simulink library "aerolibgravity2"  (Simulink 6.0)
settings: Solver=ode45  SolverMode=SingleTasking  StartTime=0.0  StopTime=10.0  RelTol=1e-3
values from neighbouring files (symbols this model uses):
  s = aeroliblist    [asbhelp.m]
undefined symbols (not defined in the file or in its folder): aeroassertmsg, c, cd, epoch, fm, fn, k, m, maxdef, snorm
libraries: simulink x9, aerolibconvert x8, aerolibutil x2
(part 2 of 2)

== system aerolibgravity2/World Magnetic Model 2000/geomg1/Compute magnetic vector in spherical coordinates/For Iterator Subsystem/Time adjust the gauss coefficients ==
  n : Inport  LatchInput=off
  m : Inport  Port=2  LatchInput=off
  dt : Inport  Port=3  LatchInput=off
  Enable : EnablePort
  Assignment : Assignment  InputType=Matrix  RowSrc=External  ColumnSrc=External  DiagnosticForDimensions=Error
  Bus Creator : BusCreator  DialogController=Simulink.DDGSource_Bus  Inputs=5
  Bus Selector1 : BusSelector  DialogController=Simulink.DDGSource_Bus  OutputSignals=signal1,signal2,signal3,signal4,signal5
  Demux2 : Demux  Outputs=3
  If Action Subsystem : Subsystem  TreatAsAtomicUnit=on  PropExecContextAcrossSSBoundary=on
  Mux1 : Mux  Inputs=3
  Sum2 : Sum  Inputs=|++  SaturateOnIntegerOverflow=on
  Unit Delay : UnitDelay  Orientation=left  X0=zeros(maxdef+1,maxdef+1)  SampleTime=-1
  c[maxdef][maxdef] : Constant  Value=c
  cd[maxdef][maxdef] : Constant  Value=cd
  if (m~=0) : Subsystem  PropExecContextAcrossSSBoundary=on
  tc[13][13] : Outport
  wires:
  Sum2/1 -> tc[13][13]/1
  Unit Delay/1 -> Assignment/1
  if (m~=0)/1(tc[13][13]) -> Sum2/2
  Bus Selector1/4 -> If Action Subsystem/4(c)  "<signal4>"
  Bus Creator/1 -> Bus Selector1/1, if (m~=0)/1(bus)
  Demux2/3 -> Assignment/4
  Demux2/2 -> Assignment/3
  Demux2/1 -> Assignment/2
  Mux1/1 -> Demux2/1
  If Action Subsystem/3(col) -> Mux1/3
  If Action Subsystem/2(row) -> Mux1/2
  If Action Subsystem/1(tc) -> Mux1/1
  Assignment/1 -> Sum2/1, Unit Delay/1
  cd[maxdef][maxdef]/1 -> Bus Creator/5
  c[maxdef][maxdef]/1 -> Bus Creator/4
  dt/1 -> Bus Creator/3
  n/1 -> Bus Creator/2
  Bus Selector1/5 -> If Action Subsystem/5(cd)  "<signal5>"
  Bus Selector1/3 -> If Action Subsystem/3(dt)  "<signal3>"
  Bus Selector1/2 -> If Action Subsystem/2(n)  "<signal2>"
  Bus Selector1/1 -> If Action Subsystem/1(m)  "<signal1>"
  m/1 -> Bus Creator/1

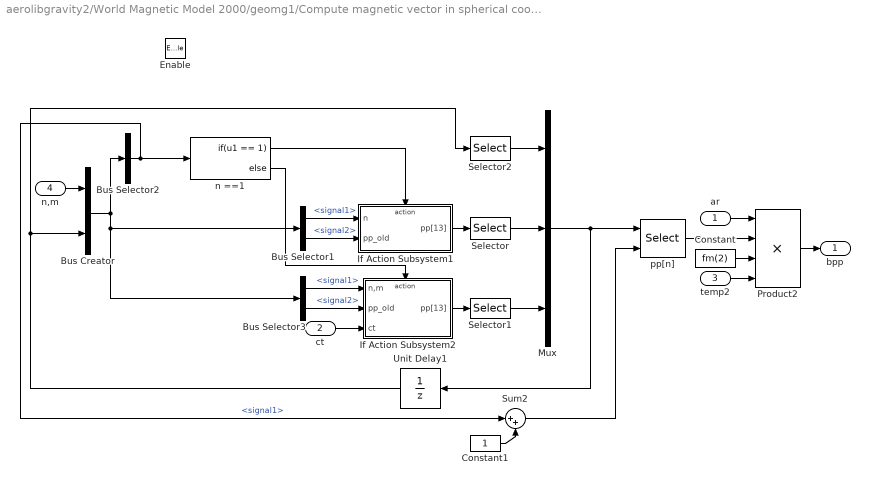
== system aerolibgravity2/World Magnetic Model 2000/geomg1/Compute magnetic vector in spherical coordinates/For Iterator Subsystem/Accumulate terms of the  spherical harmonic expansion/Special case - North/South Geographic Pole ==
  ar : Inport  LatchInput=off
  ct : Inport  Port=2  LatchInput=off
  temp2 : Inport  Port=3  LatchInput=off
  n,m : Inport  Port=4  LatchInput=off
  Enable : EnablePort
  Bus Creator : BusCreator  DialogController=Simulink.DDGSource_Bus  Inputs=2
  Bus Selector1 : BusSelector  DialogController=Simulink.DDGSource_Bus  OutputSignals=signal1.signal1,signal2
  Bus Selector2 : BusSelector  DialogController=Simulink.DDGSource_Bus  OutputSignals=signal1.signal1
  Bus Selector3 : BusSelector  DialogController=Simulink.DDGSource_Bus  OutputSignals=signal1,signal2
  Constant : Constant  Value=fm(2)
  Constant1 : Constant
  If Action Subsystem1 : Subsystem  AncestorBlock=|  PropExecContextAcrossSSBoundary=on
      | aerolibatmosratios/WMM 2000/geomg1/Compute magnetic vector in
      | spherical coordinates/For Iterator
      | Subsystem/Accumulate terms of the 
      | spherical harmonic expansion/Special case - North//South Geographic Pole/if (m~=0)/If Action
      | Subsystem1
  If Action Subsystem2 : Subsystem  AncestorBlock=|  PropExecContextAcrossSSBoundary=on
      | aerolibatmosratios/WMM 2000/geomg1/Compute magnetic vector in
      | spherical coordinates/For Iterator
      | Subsystem/Accumulate terms of the 
      | spherical harmonic expansion/Special case - North//South Geographic Pole/if (m~=0)/If Action
      | Subsystem2
  Mux : Mux  Inputs=3
  Product2 : Product  Inputs=4  SaturateOnIntegerOverflow=on
  Selector : Selector  Elements=[2]  Rows=[1 2]  Columns=-1  InputPortWidth=maxdef+1
  Selector1 : Selector  Elements=3:maxdef+1  InputPortWidth=maxdef+1
  Selector2 : Selector  Elements=[1]  Rows=[1 2]  Columns=-1  InputPortWidth=maxdef+1
  Sum2 : Sum  Inputs=|++  SaturateOnIntegerOverflow=on
  Unit Delay1 : UnitDelay  Orientation=left  X0=ones(1,maxdef+1)  SampleTime=-1
  n ==1 : If  IfExpression=u1 == 1
  pp[n] : Selector  ElementSrc=External  Elements=[1 3]  RowSrc=External  ColumnSrc=External  InputPortWidth=maxdef+1
  bpp : Outport  OutputWhenDisabled=reset  InitialOutput=0
  wires:
  Constant1/1 -> Sum2/2
  Sum2/1 -> pp[n]/2
  pp[n]/1 -> Product2/2
  Product2/1 -> bpp/1
  temp2/1 -> Product2/4
  Constant/1 -> Product2/3
  Bus Selector3/2 -> If Action Subsystem2/2(pp_old)  "<signal2>"
  Bus Selector3/1 -> If Action Subsystem2/1(n,m)  "<signal1>"
  Bus Selector1/2 -> If Action Subsystem1/2(pp_old)  "<signal2>"
  Bus Selector1/1 -> If Action Subsystem1/1(n)  "<signal1>"
  Unit Delay1/1 -> Bus Creator/2, Selector2/1
  ct/1 -> If Action Subsystem2/3(ct)
  n ==1/2 -> If Action Subsystem2/Action
  n ==1/1 -> If Action Subsystem1/Action
  If Action Subsystem2/1(pp[13]) -> Selector1/1
  If Action Subsystem1/1(pp[13]) -> Selector/1
  Bus Selector2/1 -> Sum2/1, n ==1/1  "<signal1>"
  Bus Creator/1 -> Bus Selector3/1, Bus Selector1/1, Bus Selector2/1
  ar/1 -> Product2/1
  n,m/1 -> Bus Creator/1
  Mux/1 -> Unit Delay1/1, pp[n]/1
  Selector/1 -> Mux/2
  Selector1/1 -> Mux/3
  Selector2/1 -> Mux/1

== system aerolibgravity2/World Magnetic Model 2000/geomg1/Compute magnetic vector in spherical coordinates/For Iterator Subsystem/Accumulate terms of the  spherical harmonic expansion/calculate  index ==
  n,m : Inport  LatchInput=off
  Constant : Constant
  Demux8 : Demux  Outputs=2
  Gain : Gain  Gain=maxdef+1  SaturateOnIntegerOverflow=on
  Sum1 : Sum  Inputs=+++  SaturateOnIntegerOverflow=on
  e : Outport
  wires:
  Constant/1 -> Sum1/1
  Sum1/1 -> e/1
  n,m/1 -> Demux8/1
  Demux8/2 -> Gain/1
  Demux8/1 -> Sum1/2
  Gain/1 -> Sum1/3

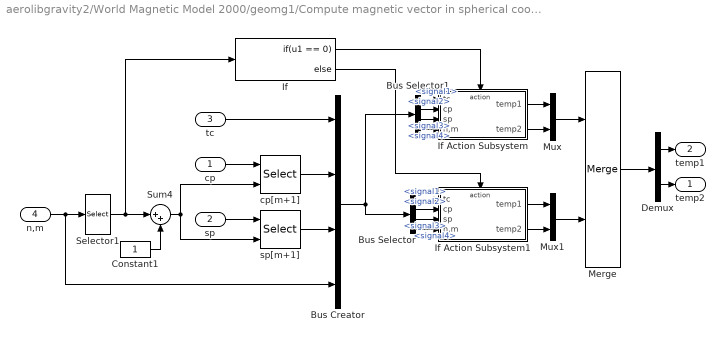
== system aerolibgravity2/World Magnetic Model 2000/geomg1/Compute magnetic vector in spherical coordinates/For Iterator Subsystem/Accumulate terms of the  spherical harmonic expansion/calculate temp values ==
  cp : Inport  LatchInput=off
  sp : Inport  Port=2  LatchInput=off
  tc : Inport  Port=3  LatchInput=off
  n,m : Inport  Port=4  LatchInput=off
  Bus Creator : BusCreator  DialogController=Simulink.DDGSource_Bus
  Bus Selector : BusSelector  DialogController=Simulink.DDGSource_Bus  OutputSignals=signal1,signal2,signal3,signal4
  Bus Selector1 : BusSelector  DialogController=Simulink.DDGSource_Bus  OutputSignals=signal1,signal2,signal3,signal4
  Constant1 : Constant
  Demux : Demux  Outputs=2
  If : If  IfExpression=u1 == 0
  If Action Subsystem : Subsystem  TreatAsAtomicUnit=on  PropExecContextAcrossSSBoundary=on
  If Action Subsystem1 : Subsystem  TreatAsAtomicUnit=on  PropExecContextAcrossSSBoundary=on
  Merge : Merge
  Mux : Mux  Inputs=2
  Mux1 : Mux  Inputs=2
  Selector1 : Selector  Elements=2  InputPortWidth=2
  Sum4 : Sum  Inputs=|++  SaturateOnIntegerOverflow=on
  cp[m+1] : Selector  ElementSrc=External  Elements=[1 3]  InputPortWidth=maxdef+1
  sp[m+1] : Selector  ElementSrc=External  Elements=[1 3]  InputPortWidth=maxdef+1
  temp2 : Outport
  temp1 : Outport  Port=2
  wires:
  Bus Selector/4 -> If Action Subsystem1/4(n,m)  "<signal4>"
  Bus Selector1/4 -> If Action Subsystem/4(n,m)  "<signal4>"
  Bus Creator/1 -> Bus Selector1/1, Bus Selector/1
  sp[m+1]/1 -> Bus Creator/3
  cp[m+1]/1 -> Bus Creator/2
  tc/1 -> Bus Creator/1
  Mux1/1 -> Merge/2
  Mux/1 -> Merge/1
  If Action Subsystem1/2(temp2) -> Mux1/2
  If Action Subsystem1/1(temp1) -> Mux1/1
  If Action Subsystem/2(temp2) -> Mux/2
  If Action Subsystem/1(temp1) -> Mux/1
  Merge/1 -> Demux/1
  Demux/2 -> temp2/1
  Demux/1 -> temp1/1
  Bus Selector/3 -> If Action Subsystem1/3(sp)  "<signal3>"
  Bus Selector/2 -> If Action Subsystem1/2(cp)  "<signal2>"
  Bus Selector/1 -> If Action Subsystem1/1(tc)  "<signal1>"
  If/2 -> If Action Subsystem1/Action
  Bus Selector1/3 -> If Action Subsystem/3(sp)  "<signal3>"
  Bus Selector1/2 -> If Action Subsystem/2(cp)  "<signal2>"
  Bus Selector1/1 -> If Action Subsystem/1(tc)  "<signal1>"
  If/1 -> If Action Subsystem/Action
  n,m/1 -> Bus Creator/4, Selector1/1
  Sum4/1 -> cp[m+1]/2, sp[m+1]/2
  Constant1/1 -> Sum4/2
  Selector1/1 -> If/1, Sum4/1
  cp/1 -> cp[m+1]/1
  sp/1 -> sp[m+1]/1

== system aerolibgravity2/World Magnetic Model 2000/geomg1/Compute magnetic vector in spherical coordinates/For Iterator Subsystem/Accumulate terms of the  spherical harmonic expansion/special case ==
  n,m : Inport  LatchInput=off
  st : Inport  Port=2  LatchInput=off
  Constant : Constant
  Constant1 : Constant  Value=0
  Logical Operator : Logic  AllPortsSameDT=off
  Relational Operator : RelationalOperator  Operator===
  Relational Operator1 : RelationalOperator  Operator===
  Selector2 : Selector  Elements=2  InputPortWidth=2
  event_sc : Outport
  wires:
  Relational Operator/1 -> Logical Operator/2
  Relational Operator1/1 -> Logical Operator/1
  Constant1/1 -> Relational Operator1/2
  Constant/1 -> Relational Operator/1
  st/1 -> Relational Operator1/1
  Logical Operator/1 -> event_sc/1
  Selector2/1 -> Relational Operator/2
  n,m/1 -> Selector2/1

== system aerolibgravity2/World Magnetic Model 2000/geomg1/Compute magnetic vector in spherical coordinates/For Iterator Subsystem/Compute unnormalized associated  legendre polynomials and  derivatives via recursion relations/If Action Subsystem ==
  snorm[169]_old : Inport  LatchInput=off
  dp[13][13]_old : Inport  Port=2  LatchInput=off
  st : Inport  Port=3  LatchInput=off
  ct : Inport  Port=4  LatchInput=off
  n,m : Inport  Port=5  LatchInput=off
  Action Port : ActionPort
  Product : Product  SaturateOnIntegerOverflow=on
  Product1 : Product  SaturateOnIntegerOverflow=on
  Product2 : Product  SaturateOnIntegerOverflow=on
  Reshape : simulink/Math Operations/Reshape  OutputDimensionality=1-D array  OutputDimensions=[1,1]
  Selector : Selector  ElementSrc=External  Elements=[1 3]  InputPortWidth=(maxdef+1)*(maxdef+1)
  Selector1 : Selector  InputType=Matrix  ElementSrc=External  Elements=[1 3]  RowSrc=External  ColumnSrc=External  InputPortWidth=(maxdef+1)*(maxdef+1)
  Sum : Sum  Inputs=|++  SaturateOnIntegerOverflow=on
  calculate  index : Subsystem  PropExecContextAcrossSSBoundary=on
  calculate  row and column : Subsystem  PropExecContextAcrossSSBoundary=on
  snorm(n+m*13) : Outport
  dp[m][n] : Outport  Port=2
  wires:
  Reshape/1 -> Product/2
  calculate  row and column/2(n) -> Selector1/3
  Product2/1 -> Sum/1
  ct/1 -> Product2/1
  Product1/1 -> snorm(n+m*13)/1
  Selector/1 -> Product2/2, Product1/2
  Product/1 -> Sum/2
  Sum/1 -> dp[m][n]/1
  st/1 -> Product1/1, Product/1
  Selector1/1 -> Reshape/1
  calculate  row and column/1(m) -> Selector1/2
  dp[13][13]_old/1 -> Selector1/1
  snorm[169]_old/1 -> Selector/1
  calculate  index/1(e) -> Selector/2
  n,m/1 -> calculate  row and column/1(n,m), calculate  index/1(n,m)

== system aerolibgravity2/World Magnetic Model 2000/geomg1/Compute magnetic vector in spherical coordinates/For Iterator Subsystem/Compute unnormalized associated  legendre polynomials and  derivatives via recursion relations/If Action Subsystem1 ==
  snorm[169]_old : Inport  LatchInput=off
  dp[13][13]_old : Inport  Port=2  LatchInput=off
  st : Inport  Port=3  LatchInput=off
  ct : Inport  Port=4  LatchInput=off
  n,m : Inport  Port=5  LatchInput=off
  Action Port : ActionPort
  Product : Product  SaturateOnIntegerOverflow=on
  Product2 : Product  SaturateOnIntegerOverflow=on
  Product3 : Product  SaturateOnIntegerOverflow=on
  Reshape : simulink/Math Operations/Reshape  OutputDimensionality=1-D array  OutputDimensions=[1,1]
  Selector : Selector  ElementSrc=External  Elements=[1 3]  InputPortWidth=(maxdef+1)*(maxdef+1)
  Selector1 : Selector  InputType=Matrix  ElementSrc=External  Elements=[1 3]  RowSrc=External  ColumnSrc=External  InputPortWidth=(maxdef+1)*(maxdef+1)
  Sum : Sum  Inputs=|-+  SaturateOnIntegerOverflow=on
  calculate  index : Subsystem  PropExecContextAcrossSSBoundary=on
  calculate  row and column : Subsystem  PropExecContextAcrossSSBoundary=on
  snorm(n+m*13) : Outport
  dp[m][n] : Outport  Port=2
  wires:
  Reshape/1 -> Product/2
  calculate  row and column/2(n) -> Selector1/3
  calculate  row and column/1(m+1) -> Selector1/2
  Sum/1 -> dp[m][n]/1
  Product2/1 -> Sum/1
  st/1 -> Product2/1
  Product3/1 -> snorm(n+m*13)/1
  Selector/1 -> Product3/2, Product2/2
  Product/1 -> Sum/2
  ct/1 -> Product3/1, Product/1
  Selector1/1 -> Reshape/1
  dp[13][13]_old/1 -> Selector1/1
  snorm[169]_old/1 -> Selector/1
  calculate  index/1(e) -> Selector/2
  n,m/1 -> calculate  row and column/1(n,m), calculate  index/1(n,m)

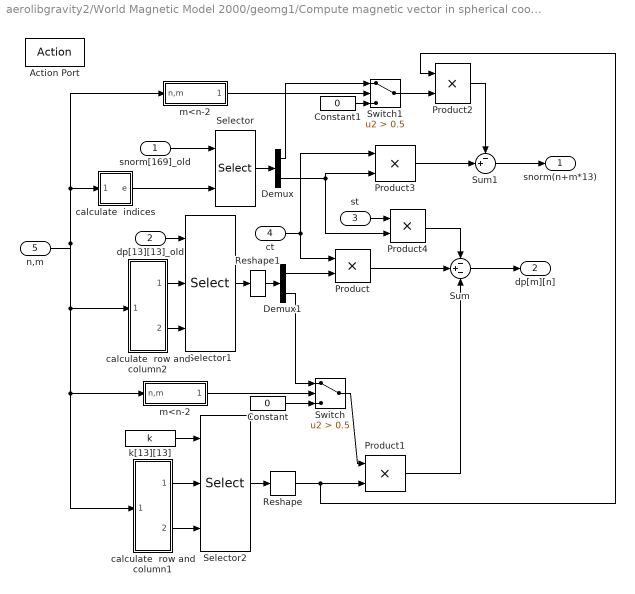
== system aerolibgravity2/World Magnetic Model 2000/geomg1/Compute magnetic vector in spherical coordinates/For Iterator Subsystem/Compute unnormalized associated  legendre polynomials and  derivatives via recursion relations/If Action Subsystem2 ==
  snorm[169]_old : Inport  LatchInput=off
  dp[13][13]_old : Inport  Port=2  LatchInput=off
  st : Inport  Port=3  LatchInput=off
  ct : Inport  Port=4  LatchInput=off
  n,m : Inport  Port=5  LatchInput=off
  Action Port : ActionPort
  Constant : Constant  Value=0
  Constant1 : Constant  Value=0
  Demux : Demux  Outputs=2
  Demux1 : Demux  Outputs=2
  Product{,1..4} (5 alike) : Product  SaturateOnIntegerOverflow=on
  Reshape : simulink/Math Operations/Reshape  OutputDimensionality=1-D array  OutputDimensions=[1,1]
  Reshape1 : simulink/Math Operations/Reshape  OutputDimensionality=1-D array  OutputDimensions=[1,1]
  Selector : Selector  ElementSrc=External  Elements=[1 3]  InputPortWidth=(maxdef+1)*(maxdef+1)
  Selector1 : Selector  InputType=Matrix  ElementSrc=External  Elements=[1 3]  RowSrc=External  ColumnSrc=External  InputPortWidth=(maxdef+1)*(maxdef+1)
  Selector2 : Selector  InputType=Matrix  ElementSrc=External  Elements=[1 3]  RowSrc=External  ColumnSrc=External  InputPortWidth=(maxdef+1)*(maxdef+1)
  Sum : Sum  Inputs=-+-  SaturateOnIntegerOverflow=on
  Sum1 : Sum  Inputs=-+|  SaturateOnIntegerOverflow=on
  Switch : Switch  Criteria=u2 > Threshold  Threshold=0.5  SaturateOnIntegerOverflow=on
  Switch1 : Switch  Criteria=u2 > Threshold  Threshold=0.5  SaturateOnIntegerOverflow=on
  calculate  indices : Subsystem  PropExecContextAcrossSSBoundary=on
  calculate  row and column1 : Subsystem  PropExecContextAcrossSSBoundary=on
  calculate  row and column2 : Subsystem  PropExecContextAcrossSSBoundary=on
  k[13][13] : Constant  Value=k
  m<n-2 : Subsystem  AncestorBlock=|  PropExecContextAcrossSSBoundary=on
      | aerolibatmosratios/WMM 2000/geomg1/Compute magnetic vector in
      | spherical coordinates/For Iterator
      | Subsystem/Compute unnormalized associated
      | legendre polynomials and
      | derivatives via recursion relations/If Action
      | Subsystem2/calculate
      | row and column
  "m<n-2 " : Subsystem  PropExecContextAcrossSSBoundary=on
  snorm(n+m*13) : Outport
  dp[m][n] : Outport  Port=2
  wires:
  "m<n-2 "/1(n-2>=m) -> Switch1/2
  Switch1/1 -> Product2/2
  Product2/1 -> Sum1/1
  Reshape1/1 -> Demux1/1
  Reshape/1 -> Product2/1, Product1/2
  Sum1/1 -> snorm(n+m*13)/1
  Constant1/1 -> Switch1/3
  Demux/1 -> Switch1/1
  Demux/2 -> Product4/2, Product3/2
  Sum/1 -> dp[m][n]/1
  m<n-2/1(n-2>=m) -> Switch/2
  Constant/1 -> Switch/3
  Switch/1 -> Product1/1
  Demux1/2 -> Switch/1
  Product1/1 -> Sum/3
  Demux1/1 -> Product/2
  Selector2/1 -> Reshape/1
  Selector/1 -> Demux/1
  calculate  row and column1/2(n+1) -> Selector2/3
  calculate  row and column1/1(m+1) -> Selector2/2
  k[13][13]/1 -> Selector2/1
  calculate  row and column2/2(n-1,n) -> Selector1/3
  calculate  row and column2/1(m+1) -> Selector1/2
  Product4/1 -> Sum/1
  st/1 -> Product4/1
  Product3/1 -> Sum1/2
  Product/1 -> Sum/2
  ct/1 -> Product3/1, Product/1
  Selector1/1 -> Reshape1/1
  dp[13][13]_old/1 -> Selector1/1
  snorm[169]_old/1 -> Selector/1
  calculate  indices/1(e) -> Selector/2
  n,m/1 -> "m<n-2 "/1(n,m), calculate  indices/1(n,m), calculate  row and column2/1(n,m), m<n-2/1(n,m), calculate  row and column1/1(n,m)

== system aerolibgravity2/World Magnetic Model 2000/geomg1/Compute magnetic vector in spherical coordinates/For Iterator Subsystem/Compute unnormalized associated  legendre polynomials and  derivatives via recursion relations/calculate  index ==
  n,m : Inport  LatchInput=off
  Constant : Constant
  Demux8 : Demux  Outputs=2
  Gain : Gain  Gain=maxdef+1  SaturateOnIntegerOverflow=on
  Sum1 : Sum  Inputs=|++  SaturateOnIntegerOverflow=on
  Sum2 : Sum  Inputs=|+-  SaturateOnIntegerOverflow=on
  e : Outport
  wires:
  Constant/1 -> Sum2/2
  Sum2/1 -> Gain/1
  Demux8/2 -> Sum2/1
  Sum1/1 -> e/1
  n,m/1 -> Demux8/1
  Demux8/1 -> Sum1/1
  Gain/1 -> Sum1/2

== system aerolibgravity2/World Magnetic Model 2000/geomg1/Compute magnetic vector in spherical coordinates/For Iterator Subsystem/Time adjust the gauss coefficients/If Action Subsystem ==
  m : Inport  LatchInput=off
  n : Inport  Port=2  LatchInput=off
  dt : Inport  Port=3  LatchInput=off
  c : Inport  Port=4  LatchInput=off
  cd : Inport  Port=5  LatchInput=off
  Constant : Constant
  Constant1 : Constant
  Product : Product  SaturateOnIntegerOverflow=on
  Sum : Sum  Inputs=|++  SaturateOnIntegerOverflow=on
  Sum1 : Sum  Inputs=|++  SaturateOnIntegerOverflow=on  InputSameDT=on
  Sum2 : Sum  Inputs=|++  SaturateOnIntegerOverflow=on  InputSameDT=on
  c[m][n] : Selector  InputType=Matrix  Elements=[1 3]  RowSrc=External  ColumnSrc=External  InputPortWidth=3
  cd[m][n] : Selector  InputType=Matrix  Elements=[1 3]  RowSrc=External  ColumnSrc=External  InputPortWidth=3
  tc : Outport
  row : Outport  Port=2
  col : Outport  Port=3
  wires:
  m/1 -> Sum1/1
  Constant1/1 -> Sum1/2
  n/1 -> Sum2/1
  Constant/1 -> Sum2/2
  Sum/1 -> tc/1
  Product/1 -> Sum/2
  c[m][n]/1 -> Sum/1
  cd[m][n]/1 -> Product/1
  dt/1 -> Product/2
  cd/1 -> cd[m][n]/1
  Sum2/1 -> cd[m][n]/3, col/1, c[m][n]/3
  Sum1/1 -> cd[m][n]/2, row/1, c[m][n]/2
  c/1 -> c[m][n]/1

== system aerolibgravity2/World Magnetic Model 2000/geomg1/Compute magnetic vector in spherical coordinates/For Iterator Subsystem/Time adjust the gauss coefficients/if (m~=0) ==
  bus : Inport  LatchInput=off
  Bus Selector : BusSelector  DialogController=Simulink.DDGSource_Bus  OutputSignals=signal1,signal2,signal3,signal4,signal5
  Bus Selector1 : BusSelector  DialogController=Simulink.DDGSource_Bus  OutputSignals=signal2
  Bus Selector2 : BusSelector  DialogController=Simulink.DDGSource_Bus  OutputSignals=signal1
  If : If  IfExpression=u1 ~= 0
  If Action Subsystem1 : Subsystem  PropExecContextAcrossSSBoundary=on
  If Action Subsystem2 : Subsystem  AncestorBlock=|  PropExecContextAcrossSSBoundary=on
      | aerolibatmosratios/WMM 2000/geomg1/Compute magnetic vector in
      | spherical coordinates/For Iterator
      | Subsystem/Time adjust the gauss coefficients/Subsystem/If Action
      | Subsystem1
  Merge : Merge
  Unit Delay : UnitDelay  Orientation=left  X0=zeros(maxdef+1,maxdef+1)  SampleTime=-1
  tc_old : Switch  Criteria=u2 > Threshold  Threshold=1  SaturateOnIntegerOverflow=on
  zeros(maxdef+1,maxdef+1) : Constant  Value=zeros(maxdef+1,maxdef+1)
  tc[13][13] : Outport
  wires:
  Unit Delay/1 -> tc_old/1
  zeros(maxdef+1,maxdef+1)/1 -> tc_old/3
  Bus Selector1/1 -> tc_old/2  "<signal2>"
  tc_old/1 -> If Action Subsystem1/6(tc_old), If Action Subsystem2/1(tc_old)
  If/2 -> If Action Subsystem2/Action
  If Action Subsystem2/1(tc[13][13]) -> Merge/2
  If Action Subsystem1/1(tc[13][13]) -> Merge/1
  Merge/1 -> Unit Delay/1, tc[13][13]/1
  bus/1 -> Bus Selector1/1, Bus Selector/1, Bus Selector2/1
  Bus Selector2/1 -> If/1  "<signal1>"
  If/1 -> If Action Subsystem1/Action
  Bus Selector/5 -> If Action Subsystem1/5(cd)  "<signal5>"
  Bus Selector/4 -> If Action Subsystem1/4(c)  "<signal4>"
  Bus Selector/3 -> If Action Subsystem1/3(dt)  "<signal3>"
  Bus Selector/2 -> If Action Subsystem1/2(n)  "<signal2>"
  Bus Selector/1 -> If Action Subsystem1/1(m)  "<signal1>"

== system aerolibgravity2/World Magnetic Model 2000/geomg1/Compute magnetic vector in spherical coordinates/For Iterator Subsystem/Accumulate terms of the  spherical harmonic expansion/Special case - North/South Geographic Pole/If Action Subsystem1 ==
  n : Inport  LatchInput=off
  pp_old : Inport  Port=2  LatchInput=off
  Action Port : ActionPort
  Assignment2 : Assignment  ElementSrc=External  RowSrc=External  ColumnSrc=External  DiagnosticForDimensions=Error
  Constant : Constant
  Sum2 : Sum  Inputs=|++  SaturateOnIntegerOverflow=on
  pp[n-1] : Selector  ElementSrc=External  Elements=[1 3]  RowSrc=External  ColumnSrc=External  InputPortWidth=maxdef+1
  pp[13] : Outport
  wires:
  pp[n-1]/1 -> Assignment2/2
  Sum2/1 -> Assignment2/3
  Constant/1 -> Sum2/2
  n/1 -> pp[n-1]/2, Sum2/1
  pp_old/1 -> pp[n-1]/1, Assignment2/1
  Assignment2/1 -> pp[13]/1

== system aerolibgravity2/World Magnetic Model 2000/geomg1/Compute magnetic vector in spherical coordinates/For Iterator Subsystem/Accumulate terms of the  spherical harmonic expansion/Special case - North/South Geographic Pole/If Action Subsystem2 ==
  n,m : Inport  LatchInput=off
  pp_old : Inport  Port=2  LatchInput=off
  ct : Inport  Port=3  LatchInput=off
  Action Port : ActionPort
  Assignment2 : Assignment  ElementSrc=External  RowSrc=External  ColumnSrc=External  DiagnosticForDimensions=Error
  Constant : Constant
  Demux8 : Demux  Outputs=2
  Product1 : Product  SaturateOnIntegerOverflow=on  InputSameDT=on
  Product2 : Product  SaturateOnIntegerOverflow=on
  Reshape : simulink/Math Operations/Reshape  OutputDimensionality=1-D array  OutputDimensions=[1,1]
  Selector1 : Selector  RowSrc=External  ColumnSrc=External  InputPortWidth=2
  Selector2 : Selector  InputType=Matrix  ElementSrc=External  Elements=[1 3]  RowSrc=External  ColumnSrc=External  InputPortWidth=(maxdef+1)*(maxdef+1)
  Sum1 : Sum  Inputs=|+-  SaturateOnIntegerOverflow=on
  Sum2 : Sum  Inputs=|++  SaturateOnIntegerOverflow=on  InputSameDT=on
  calculate  indices : Subsystem  PropExecContextAcrossSSBoundary=on
  calculate  row and column : Subsystem  PropExecContextAcrossSSBoundary=on
  k[13][13] : Constant  Value=k
  pp[n-2] pp[n-1] : Selector  ElementSrc=External  Elements=[1 3]  RowSrc=External  ColumnSrc=External  InputPortWidth=maxdef+1
  pp[13] : Outport
  wires:
  Selector1/1 -> calculate  indices/1(n), Sum2/1
  Reshape/1 -> Product1/1
  Selector2/1 -> Reshape/1
  calculate  row and column/2(n+1) -> Selector2/3
  calculate  row and column/1(m+1) -> Selector2/2
  k[13][13]/1 -> Selector2/1
  Product1/1 -> Sum1/2
  Demux8/1 -> Product1/2
  Sum1/1 -> Assignment2/2
  Product2/1 -> Sum1/1
  Demux8/2 -> Product2/2
  ct/1 -> Product2/1
  pp[n-2] pp[n-1]/1 -> Demux8/1
  calculate  indices/1(e) -> pp[n-2] pp[n-1]/2
  Assignment2/1 -> pp[13]/1
  pp_old/1 -> Assignment2/1, pp[n-2] pp[n-1]/1
  Sum2/1 -> Assignment2/3
  Constant/1 -> Sum2/2
  n,m/1 -> Selector1/1, calculate  row and column/1(n,m)

== system aerolibgravity2/World Magnetic Model 2000/geomg1/Compute magnetic vector in spherical coordinates/For Iterator Subsystem/Accumulate terms of the  spherical harmonic expansion/calculate temp values/If Action Subsystem ==
  tc : Inport  LatchInput=off
  cp : Inport  Port=2  LatchInput=off
  sp : Inport  Port=3  LatchInput=off
  n,m : Inport  Port=4  LatchInput=off
  Action Port : ActionPort
  Constant : Constant
  Demux : Demux  Outputs=2
  Demux1 : Demux  Outputs=2
  Mux : Mux  Inputs=2
  Product : Product  SaturateOnIntegerOverflow=on  InputSameDT=on
  Selector : Selector  InputType=Matrix  Elements=[1 3]  RowSrc=External  ColumnSrc=External  InputPortWidth=3
  Selector1 : Selector  Elements=[2 1]  RowSrc=External  ColumnSrc=External  InputPortWidth=2
  Sum : Sum  Inputs=|++  SaturateOnIntegerOverflow=on
  temp1 : Outport
  temp2 : Outport  Port=2
  wires:
  Demux1/2 -> temp2/1
  Demux1/1 -> temp1/1
  Product/1 -> Demux1/1
  Mux/1 -> Product/1
  Selector1/1 -> Demux/1
  Constant/1 -> Sum/2
  n,m/1 -> Sum/1
  Sum/1 -> Selector1/1
  Demux/2 -> Selector/3
  Demux/1 -> Selector/2
  Selector/1 -> Product/2
  tc/1 -> Selector/1
  sp/1 -> Mux/2
  cp/1 -> Mux/1

== system aerolibgravity2/World Magnetic Model 2000/geomg1/Compute magnetic vector in spherical coordinates/For Iterator Subsystem/Accumulate terms of the  spherical harmonic expansion/calculate temp values/If Action Subsystem1 ==
  tc : Inport  LatchInput=off
  cp : Inport  Port=2  LatchInput=off
  sp : Inport  Port=3  LatchInput=off
  n,m : Inport  Port=4  LatchInput=off
  Action Port : ActionPort
  Demux1 : Demux  Outputs=2
  Demux2 : Demux  Outputs=2
  Mux : Mux  Inputs=2
  Product : Product  SaturateOnIntegerOverflow=on  InputSameDT=on
  Product1 : Product  SaturateOnIntegerOverflow=on
  Selector : Selector  InputType=Matrix  Elements=[1 3]  RowSrc=External  ColumnSrc=External  InputPortWidth=3
  Selector1 : Selector  InputType=Matrix  Elements=[1 3]  RowSrc=External  ColumnSrc=External  InputPortWidth=3
  Sum : Sum  Inputs=|++  SaturateOnIntegerOverflow=on
  Sum1 : Sum  Inputs=|+-  SaturateOnIntegerOverflow=on
  m,n : Subsystem  PropExecContextAcrossSSBoundary=on
  n,m-1 : Subsystem  PropExecContextAcrossSSBoundary=on
  temp1 : Outport
  temp2 : Outport  Port=2
  wires:
  Demux2/1 -> Sum1/2
  Sum1/1 -> temp2/1
  Demux1/2 -> Sum1/1
  Demux2/2 -> Sum/2
  Demux1/1 -> Sum/1
  Sum/1 -> temp1/1
  Product1/1 -> Demux2/1
  Selector1/1 -> Product1/2
  n,m-1/2(col) -> Selector1/3
  n,m-1/1(row) -> Selector1/2
  Mux/1 -> Product1/1, Product/1
  sp/1 -> Mux/2
  cp/1 -> Mux/1
  n,m/1 -> n,m-1/1(n,m), m,n/1(n,m)
  m,n/2(col) -> Selector/3
  m,n/1(row) -> Selector/2
  Selector/1 -> Product/2
  tc/1 -> Selector1/1, Selector/1
  Product/1 -> Demux1/1

== system aerolibgravity2/World Magnetic Model 2000/geomg1/Compute magnetic vector in spherical coordinates/For Iterator Subsystem/Compute unnormalized associated  legendre polynomials and  derivatives via recursion relations/If Action Subsystem/calculate  index ==
  n,m : Inport  LatchInput=off
  Constant : Constant
  Demux8 : Demux  Outputs=2
  Gain : Gain  Gain=maxdef+1  SaturateOnIntegerOverflow=on
  Sum1 : Sum  Inputs=|++  SaturateOnIntegerOverflow=on
  Sum2 : Sum  Inputs=|+-  SaturateOnIntegerOverflow=on
  e : Outport
  wires:
  Constant/1 -> Sum2/2
  Sum2/1 -> Gain/1
  Sum1/1 -> e/1
  n,m/1 -> Demux8/1
  Demux8/2 -> Sum2/1
  Demux8/1 -> Sum1/1
  Gain/1 -> Sum1/2

== system aerolibgravity2/World Magnetic Model 2000/geomg1/Compute magnetic vector in spherical coordinates/For Iterator Subsystem/Compute unnormalized associated  legendre polynomials and  derivatives via recursion relations/If Action Subsystem/calculate  row and column ==
  n,m : Inport  LatchInput=off
  Demux8 : Demux  Outputs=2
  m : Outport
  n : Outport  Port=2
  wires:
  Demux8/1 -> n/1
  Demux8/2 -> m/1
  n,m/1 -> Demux8/1

== system aerolibgravity2/World Magnetic Model 2000/geomg1/Compute magnetic vector in spherical coordinates/For Iterator Subsystem/Compute unnormalized associated  legendre polynomials and  derivatives via recursion relations/If Action Subsystem1/calculate  index ==
  n,m : Inport  LatchInput=off
  Demux8 : Demux  Outputs=2
  Gain : Gain  Gain=maxdef+1  SaturateOnIntegerOverflow=on
  Sum1 : Sum  Inputs=|++  SaturateOnIntegerOverflow=on
  e : Outport
  wires:
  Sum1/1 -> e/1
  n,m/1 -> Demux8/1
  Demux8/2 -> Gain/1
  Demux8/1 -> Sum1/1
  Gain/1 -> Sum1/2

== system aerolibgravity2/World Magnetic Model 2000/geomg1/Compute magnetic vector in spherical coordinates/For Iterator Subsystem/Compute unnormalized associated  legendre polynomials and  derivatives via recursion relations/If Action Subsystem1/calculate  row and column ==
  n,m : Inport  LatchInput=off
  Constant : Constant
  Demux8 : Demux  Outputs=2
  Sum : Sum  Inputs=|++  SaturateOnIntegerOverflow=on  InputSameDT=on
  m+1 : Outport
  n : Outport  Port=2
  wires:
  Constant/1 -> Sum/2
  Sum/1 -> m+1/1
  n,m/1 -> Demux8/1
  Demux8/2 -> Sum/1
  Demux8/1 -> n/1

== system aerolibgravity2/World Magnetic Model 2000/geomg1/Compute magnetic vector in spherical coordinates/For Iterator Subsystem/Compute unnormalized associated  legendre polynomials and  derivatives via recursion relations/If Action Subsystem2/calculate  indices ==
  n,m : Inport  LatchInput=off
  Constant1 : Constant
  Demux8 : Demux  Outputs=2
  Gain : Gain  Gain=maxdef+1  SaturateOnIntegerOverflow=on
  Mux : Mux  Inputs=2
  Sum1 : Sum  Inputs=|++  SaturateOnIntegerOverflow=on
  Sum2 : Sum  Inputs=|-+  SaturateOnIntegerOverflow=on
  e : Outport
  wires:
  Mux/1 -> Sum1/1
  Sum2/1 -> Mux/1
  Constant1/1 -> Sum2/1
  Sum1/1 -> e/1
  n,m/1 -> Demux8/1
  Demux8/2 -> Gain/1
  Demux8/1 -> Mux/2, Sum2/2
  Gain/1 -> Sum1/2

== system aerolibgravity2/World Magnetic Model 2000/geomg1/Compute magnetic vector in spherical coordinates/For Iterator Subsystem/Compute unnormalized associated  legendre polynomials and  derivatives via recursion relations/If Action Subsystem2/calculate  row and column1 ==
  n,m : Inport  LatchInput=off
  Constant : Constant
  Demux8 : Demux  Outputs=2
  Sum : Sum  Inputs=|++  SaturateOnIntegerOverflow=on
  m+1 : Outport
  n+1 : Outport  Port=2
  wires:
  Sum/1 -> Demux8/1
  Constant/1 -> Sum/2
  n,m/1 -> Sum/1
  Demux8/2 -> m+1/1
  Demux8/1 -> n+1/1

== system aerolibgravity2/World Magnetic Model 2000/geomg1/Compute magnetic vector in spherical coordinates/For Iterator Subsystem/Compute unnormalized associated  legendre polynomials and  derivatives via recursion relations/If Action Subsystem2/calculate  row and column2 ==
  n,m : Inport  LatchInput=off
  Constant : Constant
  Constant1 : Constant
  Demux8 : Demux  Outputs=2
  Mux : Mux  Inputs=2
  Sum : Sum  Inputs=|++  SaturateOnIntegerOverflow=on  InputSameDT=on
  Sum2 : Sum  Inputs=|+-  SaturateOnIntegerOverflow=on
  m+1 : Outport
  n-1,n : Outport  Port=2
  wires:
  Constant/1 -> Sum/2
  Sum/1 -> m+1/1
  n,m/1 -> Demux8/1
  Demux8/2 -> Sum/1
  Demux8/1 -> Mux/1, Sum2/1
  Constant1/1 -> Sum2/2
  Sum2/1 -> Mux/2
  Mux/1 -> n-1,n/1

== system aerolibgravity2/World Magnetic Model 2000/geomg1/Compute magnetic vector in spherical coordinates/For Iterator Subsystem/Compute unnormalized associated  legendre polynomials and  derivatives via recursion relations/If Action Subsystem2/m<n-2 ==
  n,m : Inport  LatchInput=off
  Constant1 : Constant  Value=2
  Data Type Conversion : DataTypeConversion  SaturateOnIntegerOverflow=on  RndMeth=Zero
  Demux : Demux  Outputs=2
  Relational Operator : RelationalOperator
  Sum2 : Sum  Inputs=|+-  SaturateOnIntegerOverflow=on
  n-2>=m : Outport
  wires:
  Demux/2 -> Relational Operator/2
  Demux/1 -> Sum2/1
  Sum2/1 -> Relational Operator/1
  Data Type Conversion/1 -> n-2>=m/1
  n,m/1 -> Demux/1
  Constant1/1 -> Sum2/2
  Relational Operator/1 -> Data Type Conversion/1

== system aerolibgravity2/World Magnetic Model 2000/geomg1/Compute magnetic vector in spherical coordinates/For Iterator Subsystem/Compute unnormalized associated  legendre polynomials and  derivatives via recursion relations/If Action Subsystem2/m<n-2  ==
  n,m : Inport  LatchInput=off
  Constant1 : Constant  Value=2
  Data Type Conversion : DataTypeConversion  SaturateOnIntegerOverflow=on  RndMeth=Zero
  Demux : Demux  Outputs=2
  Relational Operator : RelationalOperator
  Sum2 : Sum  Inputs=|+-  SaturateOnIntegerOverflow=on
  n-2>=m : Outport
  wires:
  Demux/2 -> Relational Operator/2
  Demux/1 -> Sum2/1
  Sum2/1 -> Relational Operator/1
  Data Type Conversion/1 -> n-2>=m/1
  n,m/1 -> Demux/1
  Constant1/1 -> Sum2/2
  Relational Operator/1 -> Data Type Conversion/1

== system aerolibgravity2/World Magnetic Model 2000/geomg1/Compute magnetic vector in spherical coordinates/For Iterator Subsystem/Time adjust the gauss coefficients/if (m~=0)/If Action Subsystem1 ==
  m : Inport  LatchInput=off
  n : Inport  Port=2  LatchInput=off
  dt : Inport  Port=3  LatchInput=off
  c : Inport  Port=4  LatchInput=off
  cd : Inport  Port=5  LatchInput=off
  tc_old : Inport  Port=6  LatchInput=off
  Action Port : ActionPort
  Assignment2 : Assignment  InputType=Matrix  RowSrc=External  ColumnSrc=External  DiagnosticForDimensions=Error
  Constant : Constant
  Gain : Gain
  Product : Product  SaturateOnIntegerOverflow=on
  Sum : Sum  Inputs=|++  SaturateOnIntegerOverflow=on
  Sum2 : Sum  Inputs=|++  SaturateOnIntegerOverflow=on  InputSameDT=on
  c[m][n] : Selector  InputType=Matrix  Elements=[1 3]  RowSrc=External  ColumnSrc=External  InputPortWidth=3
  cd[m][n] : Selector  InputType=Matrix  Elements=[1 3]  RowSrc=External  ColumnSrc=External  InputPortWidth=3
  tc[13][13] : Outport
  wires:
  Assignment2/1 -> Gain/1
  tc_old/1 -> Assignment2/1
  n/1 -> Sum2/1
  Constant/1 -> Sum2/2
  m/1 -> Assignment2/4, cd[m][n]/3, c[m][n]/3
  Sum2/1 -> Assignment2/3, cd[m][n]/2, c[m][n]/2
  c/1 -> c[m][n]/1
  cd/1 -> cd[m][n]/1
  dt/1 -> Product/2
  cd[m][n]/1 -> Product/1
  c[m][n]/1 -> Sum/1
  Product/1 -> Sum/2
  Sum/1 -> Assignment2/2
  Gain/1 -> tc[13][13]/1

== system aerolibgravity2/World Magnetic Model 2000/geomg1/Compute magnetic vector in spherical coordinates/For Iterator Subsystem/Time adjust the gauss coefficients/if (m~=0)/If Action Subsystem2 ==
  tc_old : Inport  LatchInput=off
  Action Port : ActionPort
  tc[13][13] : Outport
  wires:
  tc_old/1 -> tc[13][13]/1

== system aerolibgravity2/World Magnetic Model 2000/geomg1/Compute magnetic vector in spherical coordinates/For Iterator Subsystem/Accumulate terms of the  spherical harmonic expansion/Special case - North/South Geographic Pole/If Action Subsystem2/calculate  indices ==
  n : Inport  LatchInput=off
  Constant1 : Constant
  Mux : Mux  Inputs=2
  Sum2 : Sum  Inputs=|-+  SaturateOnIntegerOverflow=on
  e : Outport
  wires:
  Mux/1 -> e/1
  Sum2/1 -> Mux/1
  Constant1/1 -> Sum2/1
  n/1 -> Mux/2, Sum2/2

== system aerolibgravity2/World Magnetic Model 2000/geomg1/Compute magnetic vector in spherical coordinates/For Iterator Subsystem/Accumulate terms of the  spherical harmonic expansion/Special case - North/South Geographic Pole/If Action Subsystem2/calculate  row and column ==
  n,m : Inport  LatchInput=off
  Constant : Constant
  Demux8 : Demux  Outputs=2
  Sum : Sum  Inputs=|++  SaturateOnIntegerOverflow=on
  m+1 : Outport
  n+1 : Outport  Port=2
  wires:
  Sum/1 -> Demux8/1
  Constant/1 -> Sum/2
  n,m/1 -> Sum/1
  Demux8/2 -> m+1/1
  Demux8/1 -> n+1/1

== system aerolibgravity2/World Magnetic Model 2000/geomg1/Compute magnetic vector in spherical coordinates/For Iterator Subsystem/Accumulate terms of the  spherical harmonic expansion/calculate temp values/If Action Subsystem1/m,n ==
  n,m : Inport  LatchInput=off
  Constant : Constant
  Demux : Demux  Outputs=2
  Selector1 : Selector  Elements=[2 1]  RowSrc=External  ColumnSrc=External  InputPortWidth=2
  Sum : Sum  Inputs=|++  SaturateOnIntegerOverflow=on
  row : Outport
  col : Outport  Port=2
  wires:
  Demux/2 -> col/1
  n,m/1 -> Sum/1
  Demux/1 -> row/1
  Selector1/1 -> Demux/1
  Constant/1 -> Sum/2
  Sum/1 -> Selector1/1

== system aerolibgravity2/World Magnetic Model 2000/geomg1/Compute magnetic vector in spherical coordinates/For Iterator Subsystem/Accumulate terms of the  spherical harmonic expansion/calculate temp values/If Action Subsystem1/n,m-1 ==
  n,m : Inport  LatchInput=off
  Constant : Constant
  Demux : Demux  Outputs=2
  Sum : Sum  Inputs=|++  SaturateOnIntegerOverflow=on
  row : Outport
  col : Outport  Port=2
  wires:
  Demux/2 -> col/1
  Sum/1 -> row/1
  Demux/1 -> Sum/1
  Constant/1 -> Sum/2
  n,m/1 -> Demux/1
